simulink model "crab_colour_track_live"  (R2019b)
settings: Solver=FixedStepAuto  StartTime=0.0  StopTime=inf  RelTol=1e-3
undefined symbols (not defined in the file): Horn, magnitude, none, Rec, Schunck, SDTV, strel, videoinput, X, Y
libraries: simulink x23, visionanalysis x6, robotlib x6, visionstatistics x4, visionmorphops x4, dspsigattribs x4, dspindex x4, raspberrypilib x4, visiontextngfix x4, visionconversions x2, dspstat3 x2, imaqlib x1
settings Model: Creator=danie  LastModifiedBy=danie
settings OptimizationCC: EnhancedBackFolding=on  PassReuseOutputArgsAs=Individual arguments  ZeroExternalMemoryAtStartup=off  ZeroInternalMemoryAtStartup=off  MaxStackSize=64  OptimizeBlockOrder=speed  DifferentSizesBufferReuse=on  OptimizationCustomize=off  EfficientTunableParamExpr=on
settings DebuggingCC: ParameterTunabilityLossMsg=error
settings HardwareCC: ProdBitPerPointer=32  ProdBitPerSizeT=32  ProdBitPerPtrDiffT=32  ProdLargestAtomicFloat=None  ProdIntDivRoundTo=Undefined  ProdEndianess=Unspecified  ProdWordSize=32  ProdHWDeviceType=Generic->Unspecified (assume 32-bit Generic)  UseEmbeddedCoderFeatures=off
settings SFSimCC: MATLABDynamicMemAlloc=off
settings RTWCC: SystemTargetFile=ert.tlc  HardwareBoard=Robot Operating System (ROS)  TLCOptions="-aInlineSetEventsForThisBaseRateFcn=TLC_FALSE -aSuppressMultiTaskScheduler=TLC_FALSE  -aRateBasedStepFcn=0"  TemplateMakefile=ert_default_tmf  GenerateReport=on  Toolchain=Catkin  IncludeHyperlinkInReport=on  LaunchReport=on  TargetLang=C++  GenerateTraceInfo=on  GenerateTraceReport=on  GenerateTraceReportSl=on  GenerateTraceReportSf=on  GenerateTraceReportEml=on
settings CodeAppCC: ForceParamTrailComments=on  IgnoreCustomStorageClasses=off  OperatorAnnotations=on  SimulinkDataObjDesc=on  SFDataObjDesc=on  InsertBlockDesc=on
settings ERTTargetCC: SupportNonInlinedSFcns=on

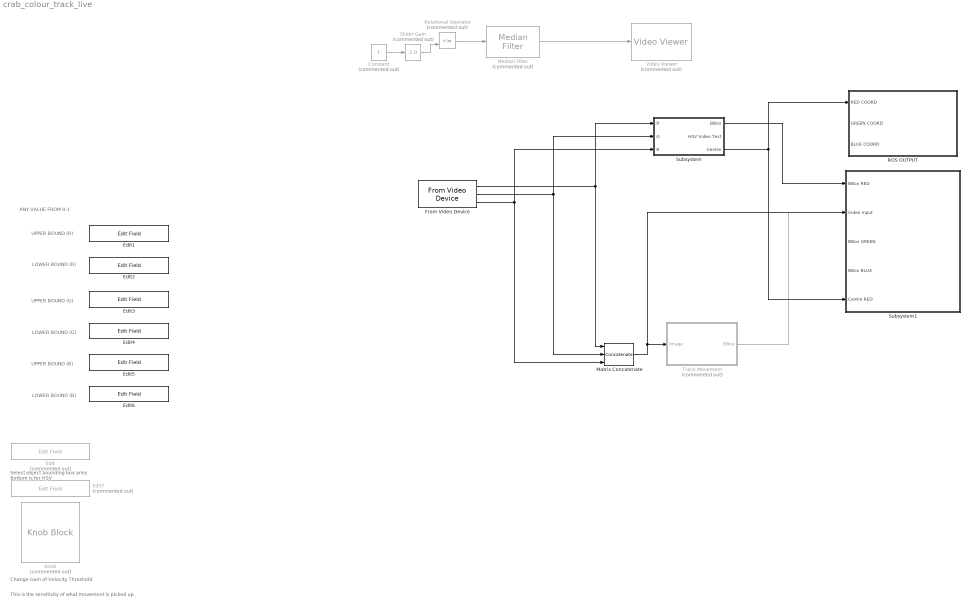
== system crab_colour_track_live ==
  note: ANY VALUE FROM 0-1
  note: Select object bounding box area
      | Bottom is for HSV
  note: LOWER BOUND (G)
  note: UPPER BOUND (R)
  note: UPPER BOUND (G)
  note: Change Gain of Velocity Threshold
  note: LOWER BOUND (R)
  note: LOWER BOUND (B)
  note: UPPER BOUND (B)
  note: This is the sensitivity of what movement is picked up
  Constant : Constant  Commented=on
  Edit : EditField  Commented=on  LabelPosition=Hide  ShowInitialText=on  Alignment=Center
  Edit{1..6} (6 alike) : EditField  LabelPosition=Hide  ShowInitialText=on  Alignment=Center
  Edit7 : EditField  Commented=on  LabelPosition=Hide  ShowInitialText=on  Alignment=Center
  From Video Device : imaqlib/From Video Device  DeviceMenu=winvideo 1 (USB_Camera)  Device=winvideo 1 (USB_Camera)  ObjConstructor=videoinput('winvideo', 1)  VideoFormatMenu=MJPG_1920x1080  VideoFormat=MJPG_1920x1080  VideoSource=input1  ROIPosition=[0 0 1080 1920]  EnableHWTrigger=off  TriggerConfiguration=none/none  SampleTime=1/30  OutputPortsMode=Separate color signals  DataType=single  CanDoHWTrigger=no  ReturnedColorSpace=rgb  BlockHandle=5428.0005  ROIWidth=1920  ROIHeight=1080  ROIColumn=0  ROIRow=0  EngXMLPath=E:\Matlab\toolbox\imaq\imaq\private  DevXMLPath=C:\ProgramData\MATLAB\SupportPackages\R2019b\toolbox\imaq\supportpackages\genericvideo\adaptor\win64  EngLibPath=E:\Matlab\toolbox\imaq\imaqblks\imaqmex\win64  ColorSpace=rgb  BayerSensorAlignment=grbg  ImaqMode=off
      settings: SourceProductName=Image Acquisition Toolbox
  Knob : KnobBlock  Commented=on
  Matrix Concatenate : Concatenate  NumInputs=3  Mode=Multidimensional array  ConcatenateDimension=3
  Median Filter : visionanalysis/Median Filter  Commented=on  nghbood=[3 3]  outSize=Same as input port I  padType=Constant  padSrc=Specify via dialog  padVal=0  roundingMode=Floor  overflowMode=off  prodOutputSlope=2^-30  accumSlope=2^-30  outputSlope=2^-15
      settings: SourceProductName=Computer Vision Toolbox  SourceProductBaseCode=VP
  ROS OUTPUT : Subsystem
  Relational Operator : RelationalOperator  Commented=on  Operator=<=  OutDataTypeStr=boolean  RndMeth=Simplest
  Slider Gain : simulink/Math Operations/Slider Gain  Commented=on  gain=2.0  low=0  high=2
  Subsystem : Subsystem
  Subsystem1 : Subsystem
  Track Movement : Subsystem  Commented=on
  Video Viewer : VideoViewer  Commented=on  FigPos=[432 922 700 548]
  wires:
  Track Movement/1(BBox) -> ?
  Relational Operator/1 -> Median Filter/1
  From Video Device/3 -> Matrix Concatenate/3, Subsystem/3(B)
  From Video Device/1 -> Matrix Concatenate/1, Subsystem/1(R)
  Constant/1 -> Slider Gain/1
  Median Filter/1 -> Video Viewer/1
  Slider Gain/1 -> Relational Operator/2
  Matrix Concatenate/1 -> Track Movement/1(Image), Subsystem1/2(Video Input)
  From Video Device/2 -> Matrix Concatenate/2, Subsystem/2(G)
  Subsystem/1(BBox) -> Subsystem1/1(BBox RED)
  Subsystem/3(Centre) -> Subsystem1/5(Centre RED), ROS OUTPUT/1(RED COORD)

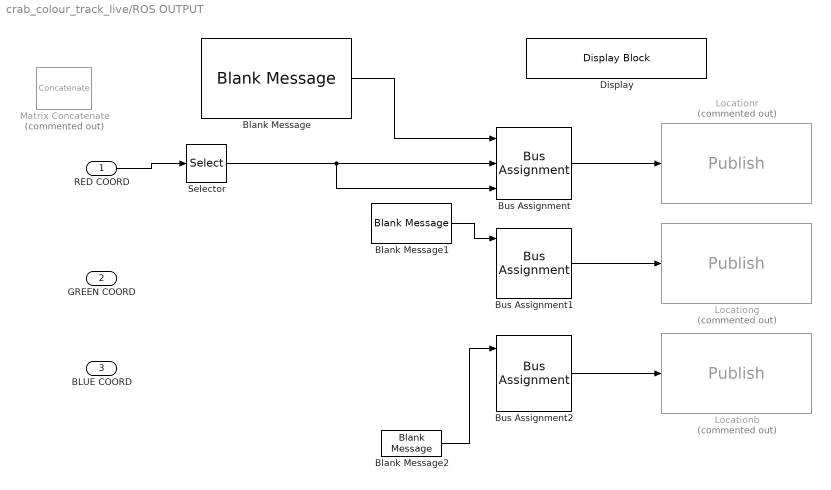
== system crab_colour_track_live/ROS OUTPUT ==
  RED COORD : Inport
  GREEN COORD : Inport  Port=2
  BLUE COORD : Inport  Port=3
  Blank Message : robotlib/Blank Message  messageClass=Message  entityType=geometry_msgs/Point  messageType=geometry_msgs/Point  SampleTime=inf
      settings: SourceProductName=ROS Toolbox
  Blank Message1 : robotlib/Blank Message  messageClass=Message  entityType=geometry_msgs/Point  messageType=geometry_msgs/Point  SampleTime=inf
      settings: SourceProductName=ROS Toolbox
  Blank Message2 : robotlib/Blank Message  messageClass=Message  entityType=geometry_msgs/Point  messageType=geometry_msgs/Point  SampleTime=inf
      settings: SourceProductName=ROS Toolbox
  Bus Assignment : BusAssignment  AssignedSignals=X,Y
  Bus Assignment1 : BusAssignment  AssignedSignals=X,Y
  Bus Assignment2 : BusAssignment  AssignedSignals=X,Y
  Display : DisplayBlock  LabelPosition=Hide  Format=short  Transparency=1
  Locationb : robotlib/Publish  Commented=on  topicSource=Specify your own  topic=/locationb  messageType=geometry_msgs/Point  messageQueueLength=1
      settings: SourceProductName=ROS Toolbox
  Locationg : robotlib/Publish  Commented=on  topicSource=Specify your own  topic=/locationg  messageType=geometry_msgs/Point  messageQueueLength=1
      settings: SourceProductName=ROS Toolbox
  Locationr : robotlib/Publish  Commented=on  topicSource=Specify your own  topic=/locationr  messageType=geometry_msgs/Point  messageQueueLength=1
      settings: SourceProductName=ROS Toolbox
  Matrix Concatenate : Concatenate  Commented=on  NumInputs=3  Mode=Multidimensional array
  Selector : Selector  NumberOfDimensions=2  InputPortWidth=3  IndexOptions=Index vector (dialog),Index vector (dialog)  Indices=1,2  OutputSizes=1,1
  wires:
  Blank Message/1 -> Bus Assignment/1
  Bus Assignment/1 -> Locationr/1
  Bus Assignment1/1 -> Locationg/1
  Bus Assignment2/1 -> Locationb/1
  Blank Message1/1 -> Bus Assignment1/1
  Blank Message2/1 -> Bus Assignment2/1
  RED COORD/1 -> Selector/1
  Selector/1 -> Bus Assignment/3, Bus Assignment/2

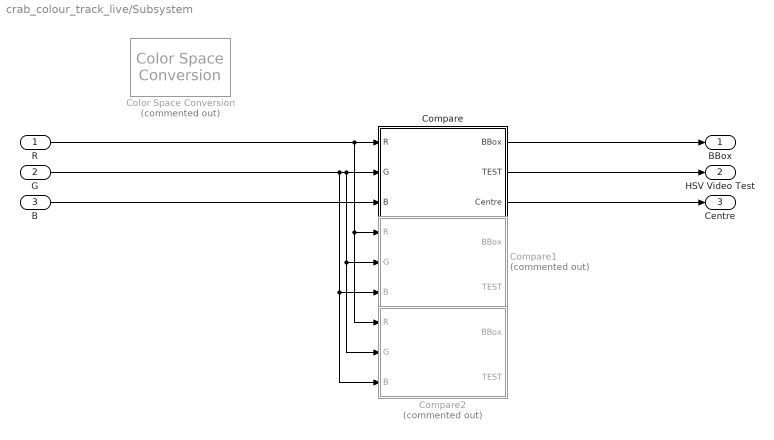
== system crab_colour_track_live/Subsystem ==
  R : Inport
  G : Inport  Port=2
  B : Inport  Port=3
  Color Space Conversion : visionconversions/Color Space  Conversion  Commented=on  conversion=Obsolete  conversionActive=R'G'B' to Y'CbCr  wp_str=D65  rec=Rec. 601 (SDTV)  sys=1125/60/2:1  imagePorts=Separate color signals
  Compare : Subsystem
  Compare1 : Subsystem  Commented=on
  Compare2 : Subsystem  Commented=on
  BBox : Outport
  HSV Video Test : Outport  Port=2
  Centre : Outport  Port=3
  wires:
  Compare/1(BBox) -> BBox/1
  Compare/2(TEST) -> HSV Video Test/1
  R/1 -> Compare2/1(R), Compare1/1(R), Compare/1(R)
  G/1 -> Compare2/3(B), Compare1/3(B), Compare2/2(G), Compare1/2(G), Compare/2(G)
  B/1 -> Compare/3(B)
  Compare/3(Centre) -> Centre/1

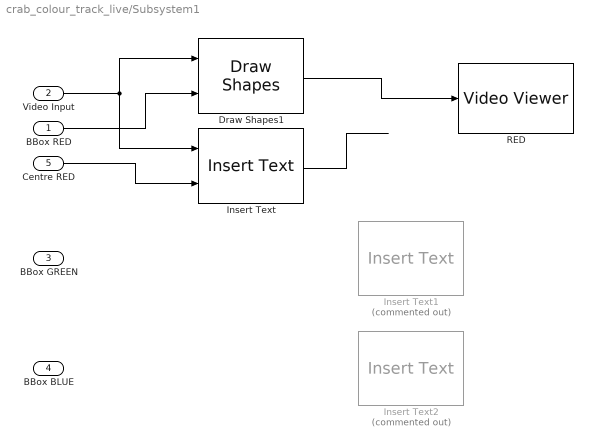
== system crab_colour_track_live/Subsystem1 ==
  BBox RED : Inport
  Video Input : Inport  Port=2
  BBox GREEN : Inport  Port=3
  BBox BLUE : Inport  Port=4
  Centre RED : Inport  Port=5
  Draw Shapes1 : visiontextngfix/Draw Shapes  shape=Rectangles  fill=off  lineWidth=1  fillClrSource=Specify via dialog  display=User-specified value  intensity=200  color=[0 255 0]  opacity=0.6  viewport=Entire image  antialiasing=off  inType=Obsolete  imagePorts=One multidimensional signal  roundingMode=Floor  overflowMode=off  memoryMode=Specify word length  memoryWordLength=16  prodOutputMode=Binary point scaling  prodOutputWordLength=32  prodOutputFracLength=14  prodOutputSlope=2^-14  accumSlope=2^-14  memoryFracLength=15
      settings: SourceProductName=Computer Vision Toolbox
  Insert Text : visiontextngfix/Insert Text  inputType=Obsolete  theText='RED'  getTextLocFrom=Input port  textLoc=[1 1]  getTextColorFrom=Specify via dialog  textColor=[0 0 0]  getTextIntensityFrom=Specify via dialog  textIntensity=0  getTextOpacityFrom=Specify via dialog  textOpacity=1.0  dummyVar2=0  dummyVar3=0  dummyVar4=0  imagePorts=One multidimensional signal  isInputTransposed=off  fontFace=LucidaSansRegular  dummyVar1=0  blockFontSize=12  antiAliased=on
      settings: SourceProductName=Computer Vision Toolbox  SourceProductBaseCode=VP
  Insert Text1 : visiontextngfix/Insert Text  Commented=on  inputType=Obsolete  theText='GREEN'  getTextLocFrom=Specify via dialog  textLoc=[1 1]  getTextColorFrom=Specify via dialog  textColor=[0 0 0]  getTextIntensityFrom=Specify via dialog  textIntensity=0  getTextOpacityFrom=Specify via dialog  textOpacity=1.0  dummyVar2=0  dummyVar3=0  dummyVar4=0  imagePorts=One multidimensional signal  isInputTransposed=off  fontFace=LucidaSansRegular  dummyVar1=0  blockFontSize=12  antiAliased=on
      settings: SourceProductName=Computer Vision Toolbox  SourceProductBaseCode=VP
  Insert Text2 : visiontextngfix/Insert Text  Commented=on  inputType=Obsolete  theText='BLUE'  getTextLocFrom=Specify via dialog  textLoc=[1 1]  getTextColorFrom=Specify via dialog  textColor=[0 0 0]  getTextIntensityFrom=Specify via dialog  textIntensity=0  getTextOpacityFrom=Specify via dialog  textOpacity=1.0  dummyVar2=0  dummyVar3=0  dummyVar4=0  imagePorts=One multidimensional signal  isInputTransposed=off  fontFace=LucidaSansRegular  dummyVar1=0  blockFontSize=12  antiAliased=on
      settings: SourceProductName=Computer Vision Toolbox  SourceProductBaseCode=VP
  RED : VideoViewer  FigPos=[962 1037 958 929]
  wires:
  Video Input/1 -> Insert Text/1, Draw Shapes1/1
  BBox RED/1 -> Draw Shapes1/2
  Centre RED/1 -> Insert Text/2
  Insert Text/1 -> ?
  Draw Shapes1/1 -> RED/1

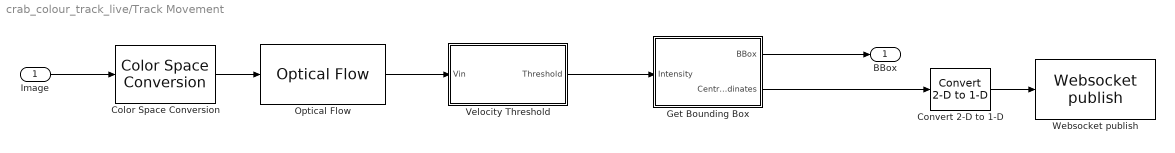
== system crab_colour_track_live/Track Movement ==
  Image : Inport
  Color Space Conversion : visionconversions/Color Space  Conversion  conversion=Obsolete  conversionActive=R'G'B' to intensity  wp_str=D65  rec=Rec. 601 (SDTV)  sys=1125/60/2:1  imagePorts=One multidimensional signal
  Convert 2-D to 1-D : dspsigattribs/Convert 2-D to 1-D
      settings: SourceProductName=DSP System Toolbox  SourceProductBaseCode=DS
  Get Bounding Box : Subsystem
  Optical Flow : visionanalysis/Optical Flow  method=Horn-Schunck  gradMethod=Difference filter [-1 1]  which2img=Current frame and N-th frame back  N=1  lambda=1  numInports=3  sigmaS=1.5  sigmaW=1  discardNormalFlow=off  outputCurrentImage=off  stop_criteria=When maximum number of iterations is reached  maxIter=10  maxAllowAbsDiff=eps  outVelForm=Horizontal and vertical components in complex form  eigTh=0.0039  roundingMode=Nearest  overflowMode=on  prodOutputMode=Binary point scaling  prodOutputWordLength=32  prodOutputFracLength=20  prodOutputSlope=2^-20  accumSlope=2^-20  memorySlope=2^-20  firstCoeffSlope=2^-20  outputMode=Binary point scaling  outputWordLength=32  outputFracLength=20  outputSlope=2^-20
      settings: SourceProductName=Computer Vision Toolbox  SourceProductBaseCode=VP
  Velocity Threshold : Subsystem
  Websocket publish : raspberrypilib/Websocket publish  UniqueBlockID=webPub 1  IPAddress=127.0.0.1  Port=9000  NumberOfSignals=1
      settings: SourceProductName=Simulink Support Package for Raspberry Pi Hardware  SourceProductBaseCode=RASPPI
  BBox : Outport
  wires:
  Image/1 -> Color Space Conversion/1
  Optical Flow/1 -> Velocity Threshold/1(Vin)
  Color Space Conversion/1 -> Optical Flow/1
  Velocity Threshold/1(Threshold) -> Get Bounding Box/1(Intensity)
  Get Bounding Box/2(Central Coordinates) -> Convert 2-D to 1-D/1
  Get Bounding Box/1(BBox) -> BBox/1
  Convert 2-D to 1-D/1 -> Websocket publish/1

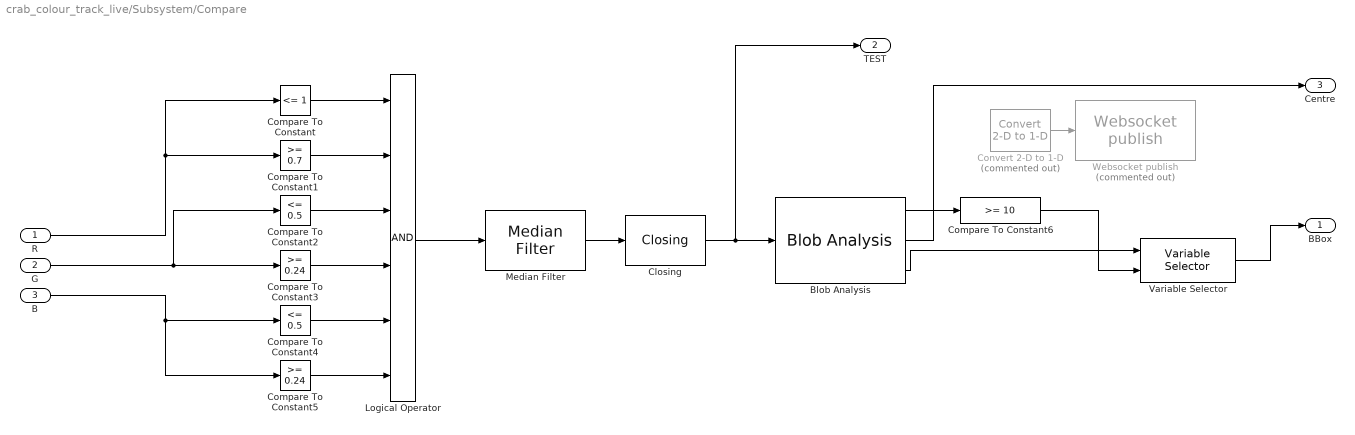
== system crab_colour_track_live/Subsystem/Compare ==
  R : Inport
  G : Inport  Port=2
  B : Inport  Port=3
  Blob Analysis : visionstatistics/Blob Analysis  Tag=vipblks_row_conv  area=on  centroid=on  bBox=on  majorAxis=off  minorAxis=off  angle=off  eccentricity=off  equivDiameterSq=off  extent=off  perimeter=off  outDT=double  conn=8  isLabel=off  maxBlobs=25  warnIfNumBlobsExceeded=on  isCount=off  useMinArea=off  minArea=0  useMaxArea=off  maxArea=intmax('uint32')  excludeBorderBlob=off  isOutVarDim=off  isFill=on  fillValues=-1  roundingMode=Floor  overflowMode=off  prodOutputMode=Binary point scaling  prodOutputWordLength=32  prodOutputFracLength=16  prodOutputSlope=2^-16  accumMode=Binary point scaling  accumWordLength=32  accumFracLength=0  accumSlope=2^0  outputMode=Binary point scaling  outputWordLength=32  outputFracLength=16  outputSlope=2^-16  memorySlope=2^-16  firstCoeffMode=Binary point scaling  firstCoeffWordLength=16  firstCoeffFracLength=14  firstCoeffSlope=2^-14  secondCoeffMode=Binary point scaling  secondCoeffWordLength=32  secondCoeffFracLength=16  secondCoeffSlope=2^-16
      settings: SourceProductName=Computer Vision Toolbox
  Closing : visionmorphops/Closing  nhoodsrc=Specify via dialog  strel=strel('line',5,45)
      settings: SourceProductName=Computer Vision Toolbox  SourceProductBaseCode=VP
  Compare To Constant : simulink/Logic and Bit Operations/Compare To Constant  relop=<=  const=1  OutDataTypeStr=boolean
  Compare To Constant1 : simulink/Logic and Bit Operations/Compare To Constant  relop=>=  const=0.7  OutDataTypeStr=boolean
  Compare To Constant2 : simulink/Logic and Bit Operations/Compare To Constant  relop=<=  const=0.5  OutDataTypeStr=boolean
  Compare To Constant3 : simulink/Logic and Bit Operations/Compare To Constant  relop=>=  const=0.24  OutDataTypeStr=boolean
  Compare To Constant4 : simulink/Logic and Bit Operations/Compare To Constant  relop=<=  const=0.5  OutDataTypeStr=boolean
  Compare To Constant5 : simulink/Logic and Bit Operations/Compare To Constant  relop=>=  const=0.24  OutDataTypeStr=boolean
  Compare To Constant6 : simulink/Logic and Bit Operations/Compare To Constant  relop=>=  const=10  OutDataTypeStr=boolean
  Convert 2-D to 1-D : dspsigattribs/Convert 2-D to 1-D  Commented=on
      settings: SourceProductName=DSP System Toolbox  SourceProductBaseCode=DS
  Logical Operator : Logic  Inputs=6  AllPortsSameDT=off  OutDataTypeStr=boolean
  Median Filter : visionanalysis/Median Filter  nghbood=[3 3]  outSize=Same as input port I  padType=Constant  padSrc=Specify via dialog  padVal=0  roundingMode=Floor  overflowMode=off  prodOutputSlope=2^-30  accumSlope=2^-30  outputSlope=2^-15
      settings: SourceProductName=Computer Vision Toolbox  SourceProductBaseCode=VP
  Variable Selector : dspindex/Variable Selector  NumInputs=1  rowsOrCols=Rows  IdxMode=Variable  Elements=[1 3]  ZerOneIdxMode=One-based  errmode=Clip Index  FillMode=on  FillValues=0
  Websocket publish : raspberrypilib/Websocket publish  Commented=on  UniqueBlockID=webPub 1  IPAddress=127.0.0.1  Port=9000  NumberOfSignals=1
      settings: SourceProductName=Simulink Support Package for Raspberry Pi Hardware  SourceProductBaseCode=RASPPI
  BBox : Outport
  TEST : Outport  Port=2
  Centre : Outport  Port=3
  wires:
  Compare To Constant/1 -> Logical Operator/1
  Compare To Constant1/1 -> Logical Operator/2
  Compare To Constant2/1 -> Logical Operator/3
  Compare To Constant3/1 -> Logical Operator/4
  Compare To Constant4/1 -> Logical Operator/5
  Compare To Constant5/1 -> Logical Operator/6
  Logical Operator/1 -> Median Filter/1
  R/1 -> Compare To Constant/1, Compare To Constant1/1
  G/1 -> Compare To Constant3/1, Compare To Constant2/1
  B/1 -> Compare To Constant5/1, Compare To Constant4/1
  Blob Analysis/2 -> Centre/1
  Blob Analysis/3 -> Variable Selector/1
  Blob Analysis/1 -> Compare To Constant6/1
  Variable Selector/1 -> BBox/1
  Convert 2-D to 1-D/1 -> Websocket publish/1
  Compare To Constant6/1 -> Variable Selector/2
  Median Filter/1 -> Closing/1
  Closing/1 -> TEST/1, Blob Analysis/1

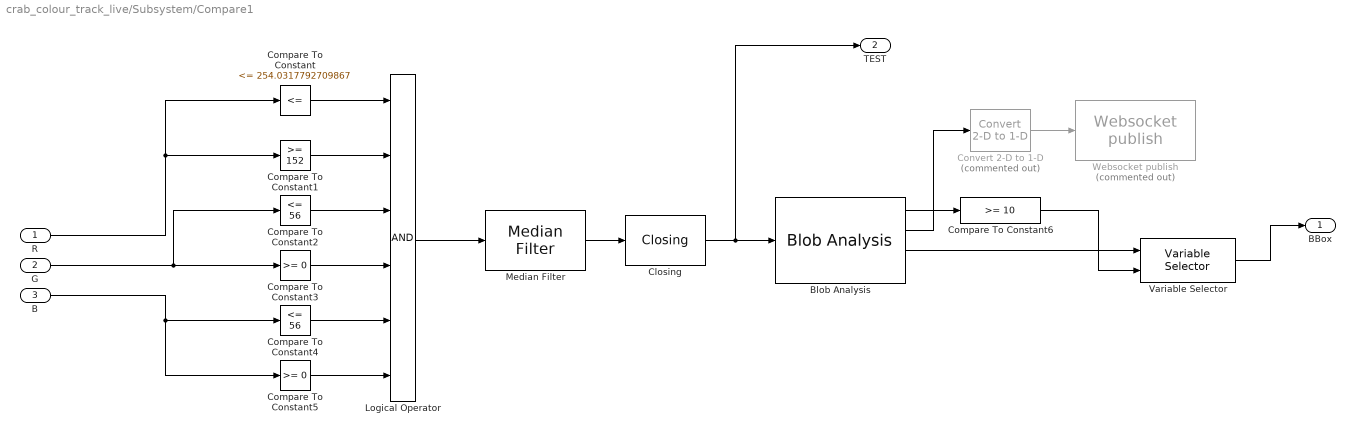
== system crab_colour_track_live/Subsystem/Compare1 ==
  R : Inport
  G : Inport  Port=2
  B : Inport  Port=3
  Blob Analysis : visionstatistics/Blob Analysis  Tag=vipblks_row_conv  area=on  centroid=on  bBox=on  majorAxis=off  minorAxis=off  angle=off  eccentricity=off  equivDiameterSq=off  extent=off  perimeter=off  outDT=double  conn=8  isLabel=on  maxBlobs=3  warnIfNumBlobsExceeded=on  isCount=off  useMinArea=off  minArea=0  useMaxArea=off  maxArea=intmax('uint32')  excludeBorderBlob=off  isOutVarDim=off  isFill=on  fillValues=-1  roundingMode=Floor  overflowMode=off  prodOutputMode=Binary point scaling  prodOutputWordLength=32  prodOutputFracLength=16  prodOutputSlope=2^-16  accumMode=Binary point scaling  accumWordLength=32  accumFracLength=0  accumSlope=2^0  outputMode=Binary point scaling  outputWordLength=32  outputFracLength=16  outputSlope=2^-16  memorySlope=2^-16  firstCoeffMode=Binary point scaling  firstCoeffWordLength=16  firstCoeffFracLength=14  firstCoeffSlope=2^-14  secondCoeffMode=Binary point scaling  secondCoeffWordLength=32  secondCoeffFracLength=16  secondCoeffSlope=2^-16
      settings: SourceProductName=Computer Vision Toolbox
  Closing : visionmorphops/Closing  nhoodsrc=Specify via dialog  strel=strel('line',5,45)
      settings: SourceProductName=Computer Vision Toolbox  SourceProductBaseCode=VP
  Compare To Constant : simulink/Logic and Bit Operations/Compare To Constant  relop=<=  const=254.0317792709867  OutDataTypeStr=boolean
  Compare To Constant1 : simulink/Logic and Bit Operations/Compare To Constant  relop=>=  const=152  OutDataTypeStr=boolean
  Compare To Constant2 : simulink/Logic and Bit Operations/Compare To Constant  relop=<=  const=56  OutDataTypeStr=boolean
  Compare To Constant3 : simulink/Logic and Bit Operations/Compare To Constant  relop=>=  const=0  OutDataTypeStr=boolean
  Compare To Constant4 : simulink/Logic and Bit Operations/Compare To Constant  relop=<=  const=56  OutDataTypeStr=boolean
  Compare To Constant5 : simulink/Logic and Bit Operations/Compare To Constant  relop=>=  const=0  OutDataTypeStr=boolean
  Compare To Constant6 : simulink/Logic and Bit Operations/Compare To Constant  relop=>=  const=10  OutDataTypeStr=boolean
  Convert 2-D to 1-D : dspsigattribs/Convert 2-D to 1-D  Commented=on
      settings: SourceProductName=DSP System Toolbox  SourceProductBaseCode=DS
  Logical Operator : Logic  Inputs=6  AllPortsSameDT=off  OutDataTypeStr=boolean
  Median Filter : visionanalysis/Median Filter  nghbood=[3 3]  outSize=Same as input port I  padType=Constant  padSrc=Specify via dialog  padVal=0  roundingMode=Floor  overflowMode=off  prodOutputSlope=2^-30  accumSlope=2^-30  outputSlope=2^-15
      settings: SourceProductName=Computer Vision Toolbox  SourceProductBaseCode=VP
  Variable Selector : dspindex/Variable Selector  NumInputs=1  rowsOrCols=Rows  IdxMode=Variable  Elements=[1 3]  ZerOneIdxMode=One-based  errmode=Clip Index  FillMode=on  FillValues=0
  Websocket publish : raspberrypilib/Websocket publish  Commented=on  UniqueBlockID=webPub 1  IPAddress=127.0.0.1  Port=9000  NumberOfSignals=1
      settings: SourceProductName=Simulink Support Package for Raspberry Pi Hardware  SourceProductBaseCode=RASPPI
  BBox : Outport
  TEST : Outport  Port=2
  wires:
  Compare To Constant/1 -> Logical Operator/1
  Compare To Constant1/1 -> Logical Operator/2
  Compare To Constant2/1 -> Logical Operator/3
  Compare To Constant3/1 -> Logical Operator/4
  Compare To Constant4/1 -> Logical Operator/5
  Compare To Constant5/1 -> Logical Operator/6
  Logical Operator/1 -> Median Filter/1
  R/1 -> Compare To Constant/1, Compare To Constant1/1
  G/1 -> Compare To Constant3/1, Compare To Constant2/1
  B/1 -> Compare To Constant5/1, Compare To Constant4/1
  Blob Analysis/2 -> Convert 2-D to 1-D/1
  Blob Analysis/3 -> Variable Selector/1
  Blob Analysis/1 -> Compare To Constant6/1
  Variable Selector/1 -> BBox/1
  Convert 2-D to 1-D/1 -> Websocket publish/1
  Compare To Constant6/1 -> Variable Selector/2
  Median Filter/1 -> Closing/1
  Closing/1 -> TEST/1, Blob Analysis/1

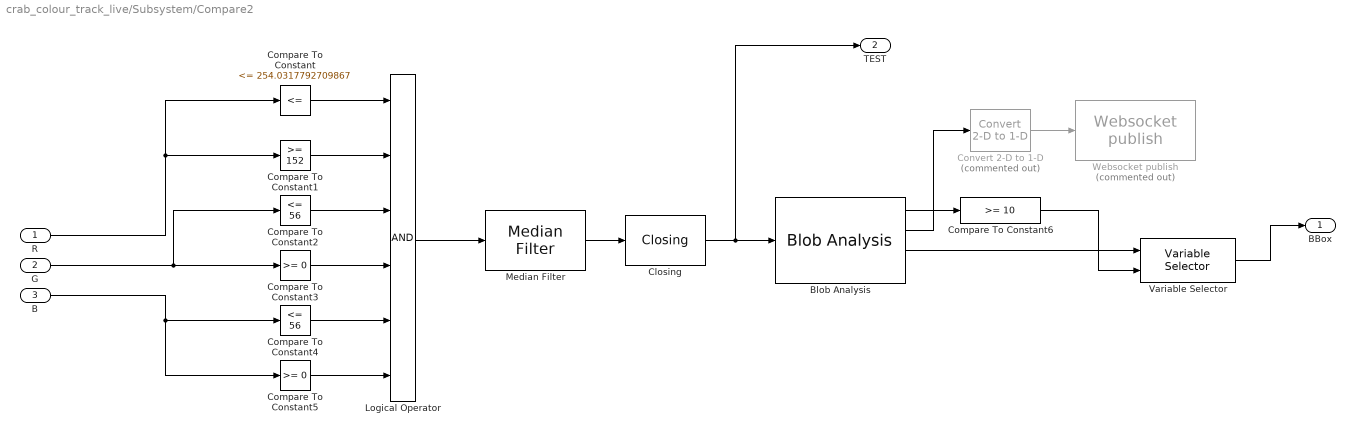
== system crab_colour_track_live/Subsystem/Compare2 ==
  R : Inport
  G : Inport  Port=2
  B : Inport  Port=3
  Blob Analysis : visionstatistics/Blob Analysis  Tag=vipblks_row_conv  area=on  centroid=on  bBox=on  majorAxis=off  minorAxis=off  angle=off  eccentricity=off  equivDiameterSq=off  extent=off  perimeter=off  outDT=double  conn=8  isLabel=on  maxBlobs=3  warnIfNumBlobsExceeded=on  isCount=off  useMinArea=off  minArea=0  useMaxArea=off  maxArea=intmax('uint32')  excludeBorderBlob=off  isOutVarDim=off  isFill=on  fillValues=-1  roundingMode=Floor  overflowMode=off  prodOutputMode=Binary point scaling  prodOutputWordLength=32  prodOutputFracLength=16  prodOutputSlope=2^-16  accumMode=Binary point scaling  accumWordLength=32  accumFracLength=0  accumSlope=2^0  outputMode=Binary point scaling  outputWordLength=32  outputFracLength=16  outputSlope=2^-16  memorySlope=2^-16  firstCoeffMode=Binary point scaling  firstCoeffWordLength=16  firstCoeffFracLength=14  firstCoeffSlope=2^-14  secondCoeffMode=Binary point scaling  secondCoeffWordLength=32  secondCoeffFracLength=16  secondCoeffSlope=2^-16
      settings: SourceProductName=Computer Vision Toolbox
  Closing : visionmorphops/Closing  nhoodsrc=Specify via dialog  strel=strel('line',5,45)
      settings: SourceProductName=Computer Vision Toolbox  SourceProductBaseCode=VP
  Compare To Constant : simulink/Logic and Bit Operations/Compare To Constant  relop=<=  const=254.0317792709867  OutDataTypeStr=boolean
  Compare To Constant1 : simulink/Logic and Bit Operations/Compare To Constant  relop=>=  const=152  OutDataTypeStr=boolean
  Compare To Constant2 : simulink/Logic and Bit Operations/Compare To Constant  relop=<=  const=56  OutDataTypeStr=boolean
  Compare To Constant3 : simulink/Logic and Bit Operations/Compare To Constant  relop=>=  const=0  OutDataTypeStr=boolean
  Compare To Constant4 : simulink/Logic and Bit Operations/Compare To Constant  relop=<=  const=56  OutDataTypeStr=boolean
  Compare To Constant5 : simulink/Logic and Bit Operations/Compare To Constant  relop=>=  const=0  OutDataTypeStr=boolean
  Compare To Constant6 : simulink/Logic and Bit Operations/Compare To Constant  relop=>=  const=10  OutDataTypeStr=boolean
  Convert 2-D to 1-D : dspsigattribs/Convert 2-D to 1-D  Commented=on
      settings: SourceProductName=DSP System Toolbox  SourceProductBaseCode=DS
  Logical Operator : Logic  Inputs=6  AllPortsSameDT=off  OutDataTypeStr=boolean
  Median Filter : visionanalysis/Median Filter  nghbood=[3 3]  outSize=Same as input port I  padType=Constant  padSrc=Specify via dialog  padVal=0  roundingMode=Floor  overflowMode=off  prodOutputSlope=2^-30  accumSlope=2^-30  outputSlope=2^-15
      settings: SourceProductName=Computer Vision Toolbox  SourceProductBaseCode=VP
  Variable Selector : dspindex/Variable Selector  NumInputs=1  rowsOrCols=Rows  IdxMode=Variable  Elements=[1 3]  ZerOneIdxMode=One-based  errmode=Clip Index  FillMode=on  FillValues=0
  Websocket publish : raspberrypilib/Websocket publish  Commented=on  UniqueBlockID=webPub 1  IPAddress=127.0.0.1  Port=9000  NumberOfSignals=1
      settings: SourceProductName=Simulink Support Package for Raspberry Pi Hardware  SourceProductBaseCode=RASPPI
  BBox : Outport
  TEST : Outport  Port=2
  wires:
  Compare To Constant/1 -> Logical Operator/1
  Compare To Constant1/1 -> Logical Operator/2
  Compare To Constant2/1 -> Logical Operator/3
  Compare To Constant3/1 -> Logical Operator/4
  Compare To Constant4/1 -> Logical Operator/5
  Compare To Constant5/1 -> Logical Operator/6
  Logical Operator/1 -> Median Filter/1
  R/1 -> Compare To Constant/1, Compare To Constant1/1
  G/1 -> Compare To Constant3/1, Compare To Constant2/1
  B/1 -> Compare To Constant5/1, Compare To Constant4/1
  Blob Analysis/2 -> Convert 2-D to 1-D/1
  Blob Analysis/3 -> Variable Selector/1
  Blob Analysis/1 -> Compare To Constant6/1
  Variable Selector/1 -> BBox/1
  Convert 2-D to 1-D/1 -> Websocket publish/1
  Compare To Constant6/1 -> Variable Selector/2
  Median Filter/1 -> Closing/1
  Closing/1 -> TEST/1, Blob Analysis/1

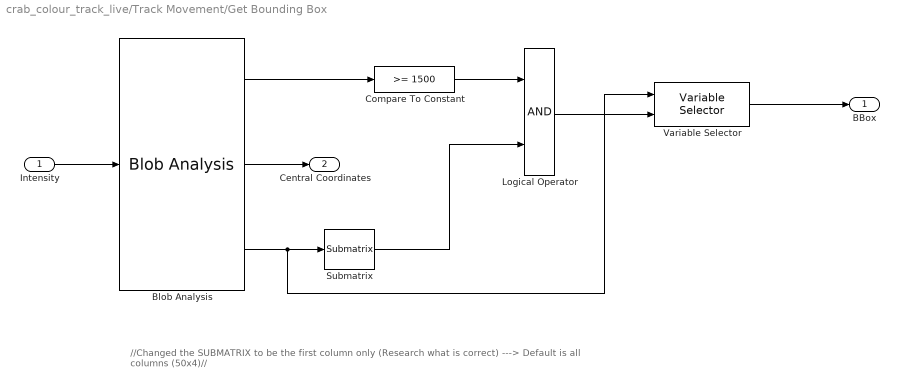
== system crab_colour_track_live/Track Movement/Get Bounding Box ==
  note: //Changed the SUBMATRIX to be the first column only (Research what is correct) ---> Default is all columns (50x4)//
  Intensity : Inport
  Blob Analysis : visionstatistics/Blob Analysis  Tag=vipblks_row_conv  area=on  centroid=on  bBox=on  majorAxis=off  minorAxis=off  angle=off  eccentricity=off  equivDiameterSq=off  extent=off  perimeter=off  outDT=double  conn=8  isLabel=off  maxBlobs=50  warnIfNumBlobsExceeded=on  isCount=off  useMinArea=off  minArea=0  useMaxArea=off  maxArea=intmax('uint32')  excludeBorderBlob=off  isOutVarDim=off  isFill=on  fillValues=-1  roundingMode=Floor  overflowMode=off  prodOutputMode=Binary point scaling  prodOutputWordLength=32  prodOutputFracLength=16  prodOutputSlope=2^-16  accumMode=Binary point scaling  accumWordLength=32  accumFracLength=0  accumSlope=2^0  outputMode=Binary point scaling  outputWordLength=32  outputFracLength=16  outputSlope=2^-16  memorySlope=2^-16  firstCoeffMode=Binary point scaling  firstCoeffWordLength=16  firstCoeffFracLength=14  firstCoeffSlope=2^-14  secondCoeffMode=Binary point scaling  secondCoeffWordLength=32  secondCoeffFracLength=16  secondCoeffSlope=2^-16
      settings: SourceProductName=Computer Vision Toolbox
  Compare To Constant : simulink/Logic and Bit Operations/Compare To Constant  relop=>=  const=1500  OutDataTypeStr=boolean
  Logical Operator : Logic  AllPortsSameDT=off  OutDataTypeStr=boolean
  Submatrix : dspmtrx3/Submatrix  RowSpan=All rows  RowStartMode=First  RowStartIndex=1  RowEndMode=Last  RowEndIndex=1  ColSpan=One column  ColStartMode=First  ColStartIndex=1  ColEndMode=Last  ColEndIndex=1
  Variable Selector : dspindex/Variable Selector  NumInputs=1  rowsOrCols=Rows  IdxMode=Variable  Elements=[1 3]  ZerOneIdxMode=One-based  errmode=Clip Index  FillMode=on  FillValues=0
  BBox : Outport
  Central Coordinates : Outport  Port=2
  wires:
  Intensity/1 -> Blob Analysis/1
  Blob Analysis/3 -> Variable Selector/1, Submatrix/1
  Compare To Constant/1 -> Logical Operator/1
  Submatrix/1 -> Logical Operator/2
  Logical Operator/1 -> Variable Selector/2
  Variable Selector/1 -> BBox/1
  Blob Analysis/2 -> Central Coordinates/1
  Blob Analysis/1 -> Compare To Constant/1

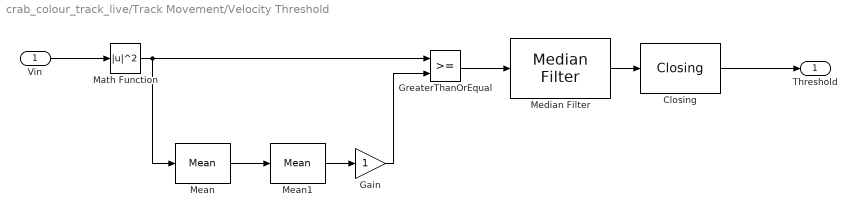
== system crab_colour_track_live/Track Movement/Velocity Threshold ==
  Vin : Inport
  Closing : visionmorphops/Closing  nhoodsrc=Specify via dialog  strel=strel('line',5,45)
      settings: SourceProductName=Computer Vision Toolbox  SourceProductBaseCode=VP
  Gain : Gain
  GreaterThanOrEqual : RelationalOperator  OutDataTypeStr=boolean  RndMeth=Simplest
  Math Function : Math  Operator=magnitude^2  SignedPower=off  SaturateOnIntegerOverflow=on
  Mean : dspstat3/Mean  run=off  InputProcessing=Columns as channels (frame based)  reset_popup=None  directionMode=Entire input  dimension=1  roiEnable=off  roiType=Rectangles  roiPortion=Entire ROI  roiOutput=Individual statistics for each ROI  roiFlag=off  roundingMode=Floor  overflowMode=off  outputDataTypeStr=Inherit: Same as accumulator  outputMin=[]  outputMax=[]  outputLastDataTypeStr=Inherit: Same as accumulator
  Mean1 : dspstat3/Mean  run=on  InputProcessing=Columns as channels (frame based)  reset_popup=None  directionMode=Each column  dimension=1  roiEnable=off  roiType=Rectangles  roiPortion=Entire ROI  roiOutput=Individual statistics for each ROI  roiFlag=off  roundingMode=Floor  overflowMode=off  outputDataTypeStr=Inherit: Same as accumulator  outputMin=[]  outputMax=[]  outputLastDataTypeStr=Inherit: Same as accumulator
  Median Filter : visionanalysis/Median Filter  nghbood=[3 3]  outSize=Same as input port I  padType=Constant  padSrc=Specify via dialog  padVal=0  roundingMode=Floor  overflowMode=off  prodOutputSlope=2^-30  accumSlope=2^-30  outputSlope=2^-15
      settings: SourceProductName=Computer Vision Toolbox  SourceProductBaseCode=VP
  Threshold : Outport
  wires:
  Vin/1 -> Math Function/1
  Math Function/1 -> Mean/1, GreaterThanOrEqual/1
  Mean/1 -> Mean1/1
  Mean1/1 -> Gain/1
  Gain/1 -> GreaterThanOrEqual/2
  GreaterThanOrEqual/1 -> Median Filter/1
  Median Filter/1 -> Closing/1
  Closing/1 -> Threshold/1
